simulink model "PID_example"  (R2020a)
settings: Solver=VariableStepAuto  StartTime=0.0  StopTime=10  RelTol=1e-3
values from neighbouring files (symbols this model uses):
  a = -3    [data_lab.mat]    (also in prgm.mat; prgm_first_lab1.m = -i)
  b = -4    [data_lab.mat]    (also in prgm.mat; prgm_first_lab1.m)
  ki = 4    [prgm.mat]
  kp = 36    [prgm.mat]
  Ts = 0.01    [data_lab.mat]    (also in prgm_first_lab1.m)
settings Model: Creator=Riyansh  LastModifiedBy=Riyansh
settings DataIOCC: ExternalInput=[t, stin]  LoadExternalInput=on  SaveFormat=Array  ReturnWorkspaceOutputs=off

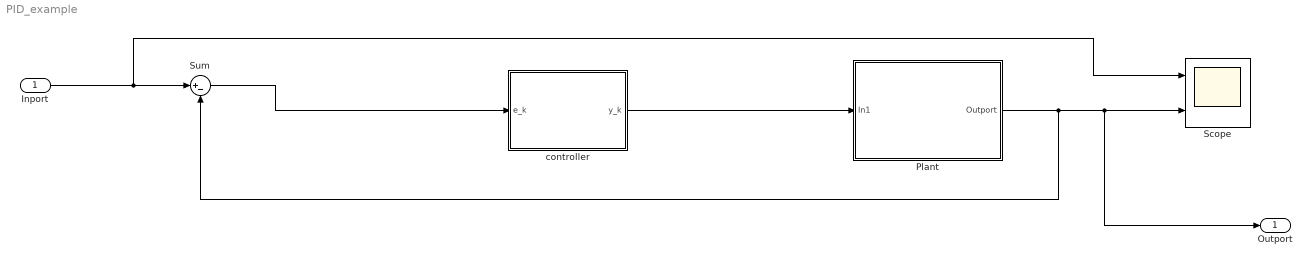
== system PID_example ==
  Inport : Inport
  Plant : Subsystem
  Scope : Scope  NumInputPorts=2
  Sum : Sum  Inputs=|+-
  controller : Subsystem
  Outport : Outport
  wires:
  Inport/1 -> Scope/1, Sum/1
  controller/1(y_k) -> Plant/1(In1)
  Plant/1(Outport) -> Sum/2, Outport/1, Scope/2
  Sum/1 -> controller/1(e_k)

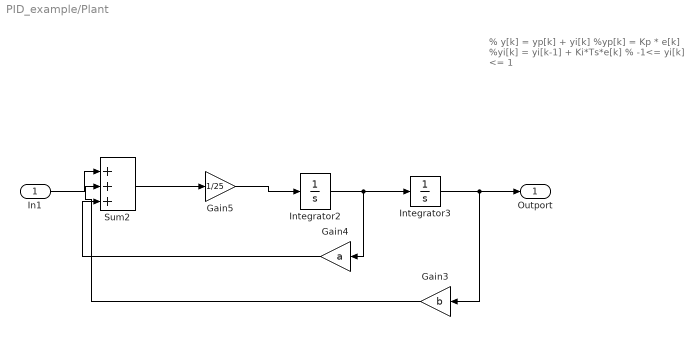
== system PID_example/Plant ==
  note: % y[k] = yp[k] + yi[k]
      |
      | %yp[k] = Kp * e[k]
      |
      | %yi[k] = yi[k-1] + Ki*Ts*e[k]
      |
      | % -1<= yi[k] <= 1
  In1 : Inport
  Gain3 : Gain  Gain=b
  Gain4 : Gain  Gain=a
  Gain5 : Gain  Gain=1/25
  Integrator2 : Integrator
  Integrator3 : Integrator
  Sum2 : Sum  Inputs=|+++
  Outport : Outport
  wires:
  Integrator3/1 -> Outport/1, Gain3/1
  In1/1 -> Sum2/1
  Gain5/1 -> Integrator2/1
  Integrator2/1 -> Gain4/1, Integrator3/1
  Sum2/1 -> Gain5/1
  Gain4/1 -> Sum2/3
  Gain3/1 -> Sum2/2

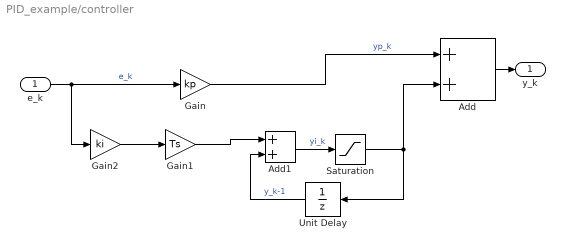
== system PID_example/controller ==
  e_k : Inport
  Add : Sum
  Add1 : Sum
  Gain : Gain  Gain=kp
  Gain1 : Gain  Gain=Ts
  Gain2 : Gain  Gain=ki
  Saturation : Saturate  UpperLimit=1  LowerLimit=-1
  Unit Delay : UnitDelay  SampleTime=-1  HasFrameUpgradeWarning=on
  y_k : Outport
  wires:
  Saturation/1 -> Add/2, Unit Delay/1
  Gain2/1 -> Gain1/1
  Unit Delay/1 -> Add1/2  "y_k-1"
  Add1/1 -> Saturation/1  "yi_k"
  Gain/1 -> Add/1  "yp_k"
  e_k/1 -> Gain2/1, Gain/1  "e_k"
  Gain1/1 -> Add1/1
  Add/1 -> y_k/1
